simulink model "sigdemo_large_STRONG_SIGNATURE"  (Simulink 8.4)
settings: Solver=FixedStepDiscrete  StartTime=0.0  StopTime=50.0  FixedStep=0.0001  RelTol=1e-3
undefined symbols (not defined in the file or in its folder): CheckValue, DefaultMode, ErrorMode, FALSE, Mode1, Mode1Cal, Mode2, Mode3, Mode3Cal, Mode4, Mode4Cal, Mode4Val, TRUE
settings Model: Creator=chrysler2  LastModifiedBy=Ben
settings DebuggingCC: CheckSSInitialOutputMsg=off  MergeDetectMultiDrivingBlocksExec=error  FcnCallInpInsideContextMsg=EnableAllAsWarning

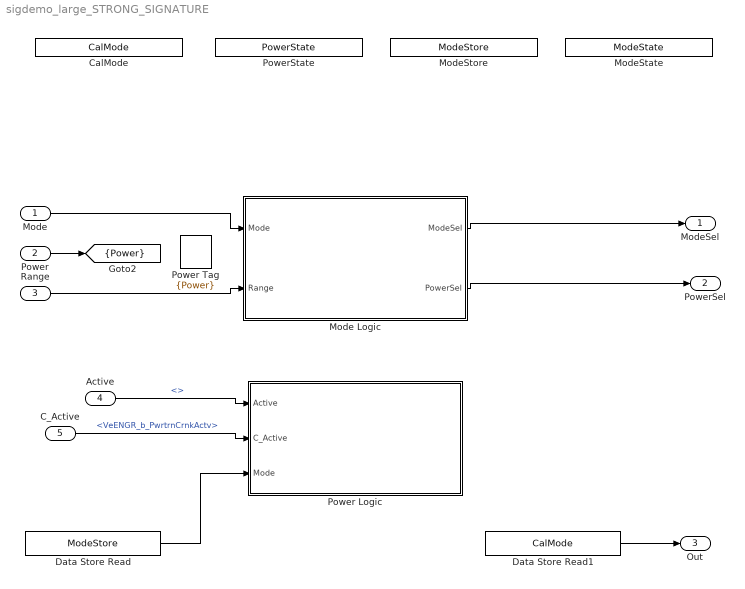
== system sigdemo_large_STRONG_SIGNATURE ==
  Mode : Inport
  Power : Inport  Port=2
  Range : Inport  Port=3
  Active : Inport  Port=4
  C_Active : Inport  Port=5
  CalMode : DataStoreMemory  DataStoreName=CalMode  OutDataTypeStr=uint16
  Data Store Read : DataStoreRead  DataStoreName=ModeStore
  Data Store Read1 : DataStoreRead  DataStoreName=CalMode
  Mode Logic : Subsystem
  ModeState : DataStoreMemory  DataStoreName=ModeState  OutDataTypeStr=uint16
  ModeStore : DataStoreMemory  DataStoreName=ModeStore  OutDataTypeStr=uint16
  Power Logic : Subsystem
  Power Tag : GotoTagVisibility  GotoTag=Power
  PowerState : DataStoreMemory  DataStoreName=PowerState  OutDataTypeStr=boolean
  ModeSel : Outport
  PowerSel : Outport  Port=2
  Out : Outport  Port=3
  tag scope: Power=scoped
  wires:
  Mode Logic/1(ModeSel) -> ModeSel/1
  Mode Logic/2(PowerSel) -> PowerSel/1
  Range/1 -> Mode Logic/2(Range)
  C_Active/1 -> Power Logic/2(C_Active)  "<VeENGR_b_PwrtrnCrnkActv>"
  Active/1 -> Power Logic/1(Active)  "<>"
  Mode/1 -> Mode Logic/1(Mode)
  Data Store Read/1 -> Power Logic/3(Mode)
  Data Store Read1/1 -> Out/1
  Power/1 -> [Power]

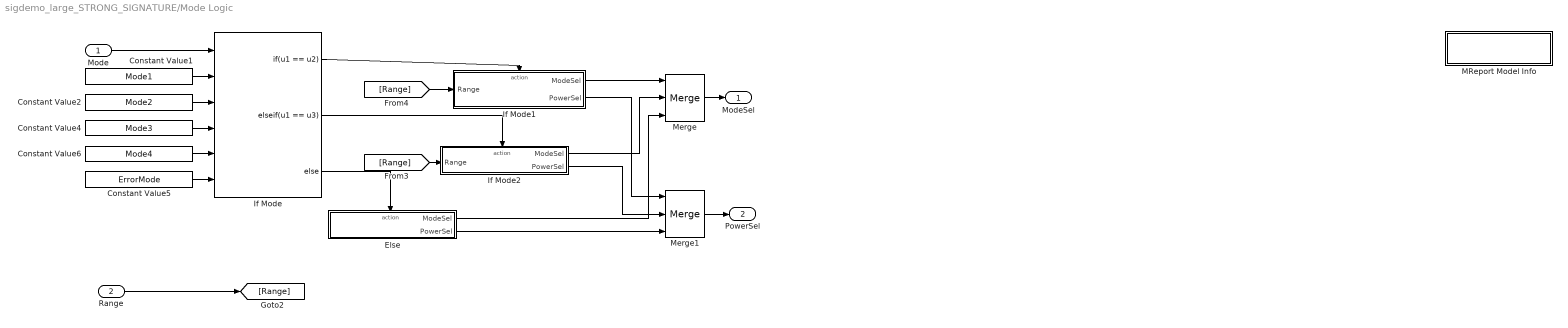
== system sigdemo_large_STRONG_SIGNATURE/Mode Logic ==
  Mode : Inport
  Range : Inport  Port=2
  Constant Value1 : Constant  Tag=R12-1  Value=Mode1  OutDataTypeStr=uint16  SampleTime=-1
  Constant Value2 : Constant  Tag=R12-1  Value=Mode2  OutDataTypeStr=uint16  SampleTime=-1
  Constant Value4 : Constant  Tag=R12-1  Value=Mode3  OutDataTypeStr=uint16  SampleTime=-1
  Constant Value5 : Constant  Tag=R12-1  Value=ErrorMode  OutDataTypeStr=uint16  SampleTime=-1
  Constant Value6 : Constant  Tag=R12-1  Value=Mode4  OutDataTypeStr=uint16  SampleTime=-1
  Else : Subsystem  TreatAsAtomicUnit=on
  If Mode : If  NumInputs=6  IfExpression=u1 == u2  ElseIfExpressions=u1 == u3
  If Mode1 : Subsystem  TreatAsAtomicUnit=on
  If Mode2 : Subsystem  TreatAsAtomicUnit=on
  MReport Model Info : Subsystem  mask(CMBlock){FollowLink=off, DocumentationField=|, HistoryField=, External=0}
      mask DocumentationField=|
      | This subsystem determines the desired neutral range state and desired engine state based on the PRNDL state.
      | The Drive functionality is executed when the PRNDL state is in DRIVE6 mode while the reverse functionality is triggered when PRNDL state is REVERSE. For other PRNDL states like Park, Neutral or Illegal the PNI functionality is executed.
      mask prompts: External "Mask Parameter 4:"
      mask help: This block allows to manage subsystem and history information.
      settings: OpenFcn=if isempty(which('mreport')),answer = char(inputdlg('Please define MReport path:'));addpath(answer);addpath([answer]);end;mr_model_info;
      mask Display: disp('MReport Model Info')
  Merge : Merge  Tag=R12-1  Inputs=3
  Merge1 : Merge  Tag=R12-1  Inputs=3
  ModeSel : Outport
  PowerSel : Outport  Port=2
  wires:
  [Range] -> If Mode2/1(Range)
  Mode/1 -> If Mode/1
  Constant Value1/1 -> If Mode/2
  Constant Value2/1 -> If Mode/3
  Constant Value4/1 -> If Mode/4
  Constant Value6/1 -> If Mode/5
  Constant Value5/1 -> If Mode/6
  If Mode/1 -> If Mode1/Action
  If Mode/3 -> Else/Action
  If Mode/2 -> If Mode2/Action
  Range/1 -> [Range]
  [Range] -> If Mode1/1(Range)
  If Mode1/1(ModeSel) -> Merge/1
  Merge/1 -> ModeSel/1
  Merge1/1 -> PowerSel/1
  If Mode1/2(PowerSel) -> Merge1/1
  If Mode2/1(ModeSel) -> Merge/2
  Else/1(ModeSel) -> Merge/3
  If Mode2/2(PowerSel) -> Merge1/2
  Else/2(PowerSel) -> Merge1/3

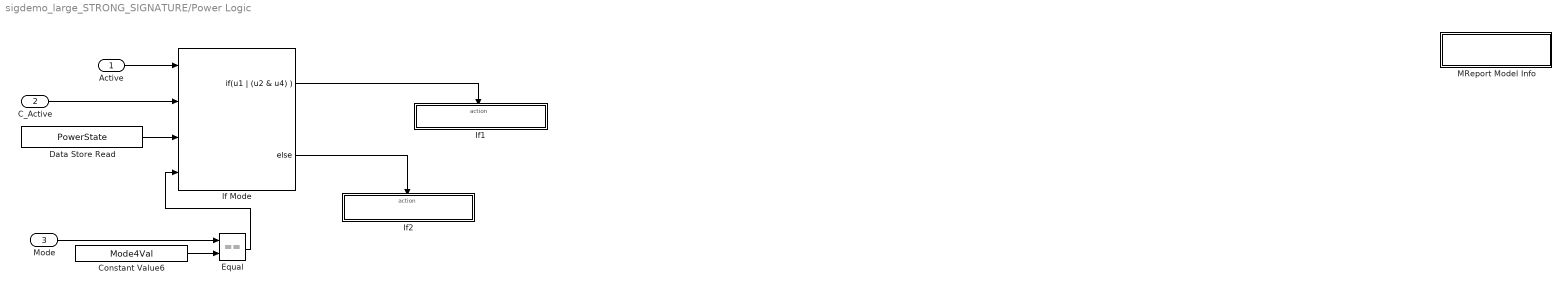
== system sigdemo_large_STRONG_SIGNATURE/Power Logic ==
  Active : Inport
  C_Active : Inport  Port=2
  Mode : Inport  Port=3
  Constant Value6 : Constant  Tag=R12-1  Value=Mode4Val  OutDataTypeStr=uint16  SampleTime=-1
  Data Store Read : DataStoreRead  DataStoreName=PowerState
  Equal : RelationalOperator  Tag=R12-1  Operator===  OutDataTypeStr=boolean  InputSameDT=on
  If Mode : If  NumInputs=4  IfExpression=u1 | (u2 & u4)
  If1 : Subsystem  TreatAsAtomicUnit=on
  If2 : Subsystem  TreatAsAtomicUnit=on
  MReport Model Info : Subsystem  mask(CMBlock){FollowLink=off, DocumentationField=|, HistoryField=, External=0}
      mask DocumentationField=|
      | This subsystem updates the following based on Gear Range state, Crank Now status, Power status and PT Active status:
      | a) Power On Timer Value
      | b) Power On Cold True Status
      | c) Power Status
      | d) Power On Cold Cost value
      |
      | The Power On functionality is triggered when PT is active or Cranking is enabled and Gear Range is in Parking or Neutral state otherwise the Power Off functionality is enabled to disable the Power status and updates Gear Range state by the Clutch Park or Neutral state. The Current Entry functionality is executed when the Power status is enabled.
      mask prompts: External "Mask Parameter 4:"
      mask help: This block allows to manage subsystem and history information.
      settings: OpenFcn=if isempty(which('mreport')),answer = char(inputdlg('Please define MReport path:'));addpath(answer);addpath([answer]);end;mr_model_info;
      mask Display: disp('MReport Model Info')
  wires:
  If Mode/2 -> If2/Action
  If Mode/1 -> If1/Action
  Active/1 -> If Mode/1
  C_Active/1 -> If Mode/2
  Data Store Read/1 -> If Mode/3
  Mode/1 -> Equal/1
  Constant Value6/1 -> Equal/2
  Equal/1 -> If Mode/4

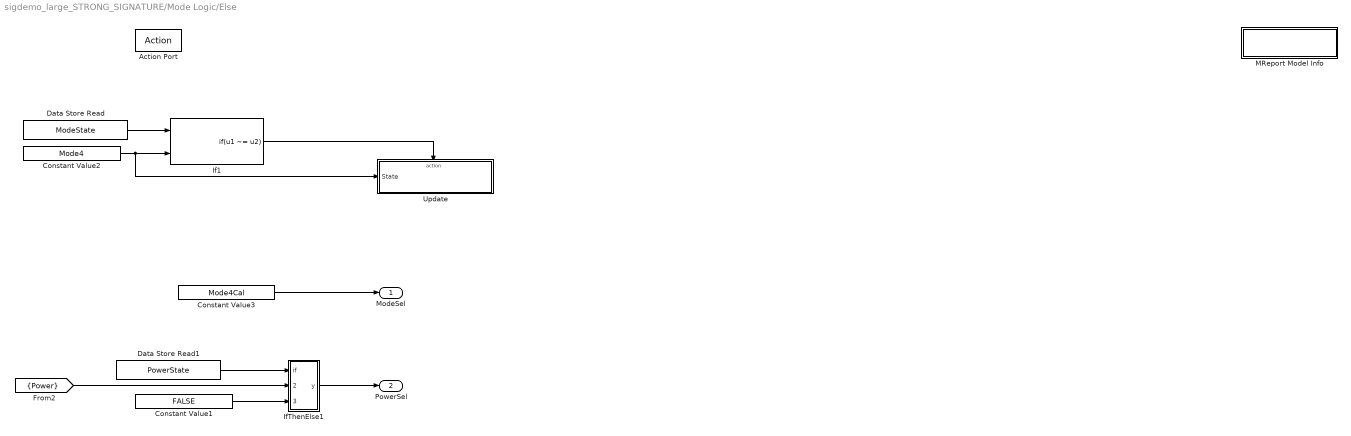
== system sigdemo_large_STRONG_SIGNATURE/Mode Logic/Else ==
  Action Port : ActionPort
  Constant Value1 : Constant  Tag=R12-1  Value=FALSE  OutDataTypeStr=boolean  SampleTime=-1
  Constant Value2 : Constant  Tag=R12-1  Value=Mode4  OutDataTypeStr=uint16  SampleTime=-1
  Constant Value3 : Constant  Tag=R12-1  Value=Mode4Cal  OutDataTypeStr=uint16  SampleTime=-1
  Data Store Read : DataStoreRead  DataStoreName=ModeState
  Data Store Read1 : DataStoreRead  DataStoreName=PowerState
  If1 : If  NumInputs=2  IfExpression=u1 ~= u2  ShowElse=off
  IfThenElse1 : Subsystem  Tag=R12-1  mask(IfElseif){}
      mask help: Output signal(s) will equal "then" values when "if" is TRUE, or hold their values if FALSE. Multiple signals can be pass by vectorizing the signals through the use of a mux block. Input1=IF condtion; Input2=IF action; Input3=ELSE action.
      mask Help: web(char(which([char(get_param(gcb,'MaskType')),'.html'])));
  MReport Model Info : Subsystem  mask(CMBlock){FollowLink=off, DocumentationField=|, HistoryField=, External=0}
      mask DocumentationField=|
      | This subsystem updates the following:
      | 1. State of Gear Range State by the PRNDL NEUTRAL state, Gear Range state by the Clutch Park or Neutral state. The Current Entry functionality is executed when the Gear Range State is not in PRNDL NEUTRAL state.
      | 2. Desired Neutral Range state by the Neutral Range Selection state.
      | 3. Desired Engine Selection indication by the Engine Selection indication or disables it depending upon Power Status.
      mask prompts: External "Mask Parameter 4:"
      mask help: This block allows to manage subsystem and history information.
      settings: OpenFcn=if isempty(which('mreport')),answer = char(inputdlg('Please define MReport path:'));addpath(answer);addpath([answer]);end;mr_model_info;
      mask Display: disp('MReport Model Info')
  Update : Subsystem  TreatAsAtomicUnit=on
  ModeSel : Outport
  PowerSel : Outport  Port=2
  wires:
  Data Store Read/1 -> If1/1
  If1/1 -> Update/Action
  Constant Value2/1 -> Update/1(State), If1/2
  IfThenElse1/1(y) -> PowerSel/1
  Data Store Read1/1 -> IfThenElse1/1(if)
  Constant Value1/1 -> IfThenElse1/3(else)
  Constant Value3/1 -> ModeSel/1
  [Power] -> IfThenElse1/2(then)

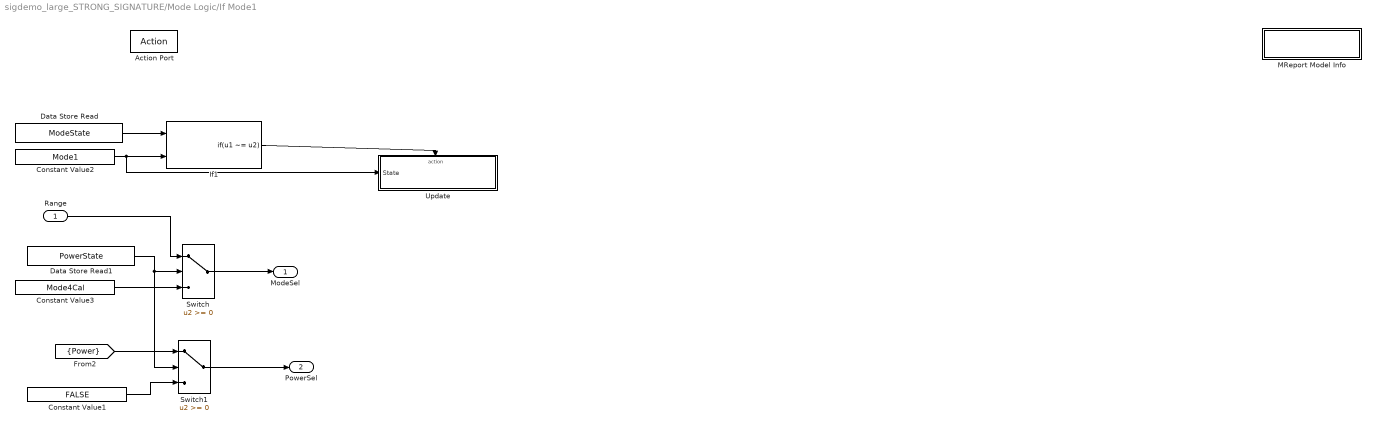
== system sigdemo_large_STRONG_SIGNATURE/Mode Logic/If Mode1 ==
  Range : Inport
  Action Port : ActionPort
  Constant Value1 : Constant  Tag=R12-1  Value=FALSE  OutDataTypeStr=boolean  SampleTime=-1
  Constant Value2 : Constant  Tag=R12-1  Value=Mode1  OutDataTypeStr=uint16  SampleTime=-1
  Constant Value3 : Constant  Tag=R12-1  Value=Mode4Cal  OutDataTypeStr=uint16  SampleTime=-1
  Data Store Read : DataStoreRead  DataStoreName=ModeState
  Data Store Read1 : DataStoreRead  DataStoreName=PowerState
  If1 : If  NumInputs=2  IfExpression=u1 ~= u2  ShowElse=off
  MReport Model Info : Subsystem  mask(CMBlock){FollowLink=off, DocumentationField=|, HistoryField=, External=0}
      mask DocumentationField=|
      | This subsystem updates the following:
      | 1. State of Gear Range State by the PRNDL DRIVE6 state and Gear Range state by the Clutch Drive state.The Current Entry functionality is executed when the Gear Range State is not in PRNDL DRIVE6 state.
      | 2. Desired Neutral Range state by the  Selection Range state or by Neutral Range Selection state based on Power Status.
      | 3. Desired Engine Selection indication by  Engine Selection indication or disables it based on Power Status.
      mask prompts: External "Mask Parameter 4:"
      mask help: This block allows to manage subsystem and history information.
      settings: OpenFcn=if isempty(which('mreport')),answer = char(inputdlg('Please define MReport path:'));addpath(answer);addpath([answer]);end;mr_model_info;
      mask Display: disp('MReport Model Info')
  Switch : Switch
  Switch1 : Switch
  Update : Subsystem  TreatAsAtomicUnit=on
  ModeSel : Outport
  PowerSel : Outport  Port=2
  wires:
  Data Store Read/1 -> If1/1
  If1/1 -> Update/Action
  Constant Value2/1 -> If1/2, Update/1(State)
  Switch/1 -> ModeSel/1
  Switch1/1 -> PowerSel/1
  Data Store Read1/1 -> Switch/2, Switch1/2
  Constant Value1/1 -> Switch1/3
  Constant Value3/1 -> Switch/3
  Range/1 -> Switch/1
  [Power] -> Switch1/1

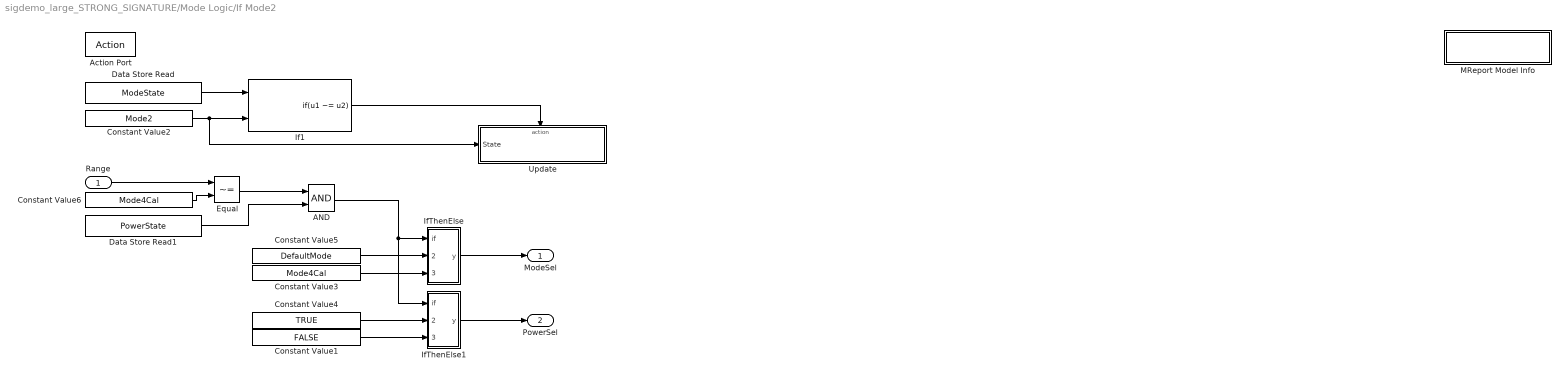
== system sigdemo_large_STRONG_SIGNATURE/Mode Logic/If Mode2 ==
  Range : Inport
  Action Port : ActionPort
  AND : Logic  Tag=R12-1  OutDataTypeStr=boolean
  Constant Value1 : Constant  Tag=R12-1  Value=FALSE  OutDataTypeStr=boolean  SampleTime=-1
  Constant Value2 : Constant  Tag=R12-1  Value=Mode2  OutDataTypeStr=uint16  SampleTime=-1
  Constant Value3 : Constant  Tag=R12-1  Value=Mode4Cal  OutDataTypeStr=uint16  SampleTime=-1
  Constant Value4 : Constant  Tag=R12-1  Value=TRUE  OutDataTypeStr=boolean  SampleTime=-1
  Constant Value5 : Constant  Tag=R12-1  Value=DefaultMode  OutDataTypeStr=uint16  SampleTime=-1
  Constant Value6 : Constant  Tag=R12-1  Value=Mode4Cal  OutDataTypeStr=uint16  SampleTime=-1
  Data Store Read : DataStoreRead  DataStoreName=ModeState
  Data Store Read1 : DataStoreRead  DataStoreName=PowerState
  Equal : RelationalOperator  Tag=R12-1  Operator=~=  OutDataTypeStr=boolean
  If1 : If  NumInputs=2  IfExpression=u1 ~= u2  ShowElse=off
  IfThenElse : Subsystem  Tag=R12-1  mask(IfElseif){}
      mask help: Output signal(s) will equal "then" values when "if" is TRUE, or hold their values if FALSE. Multiple signals can be pass by vectorizing the signals through the use of a mux block. Input1=IF condtion; Input2=IF action; Input3=ELSE action.
      mask Help: web(char(which([char(get_param(gcb,'MaskType')),'.html'])));
  IfThenElse1 : Subsystem  Tag=R12-1  mask(IfElseif){}
      mask help: Output signal(s) will equal "then" values when "if" is TRUE, or hold their values if FALSE. Multiple signals can be pass by vectorizing the signals through the use of a mux block. Input1=IF condtion; Input2=IF action; Input3=ELSE action.
      mask Help: web(char(which([char(get_param(gcb,'MaskType')),'.html'])));
  MReport Model Info : Subsystem  mask(CMBlock){FollowLink=off, DocumentationField=|, HistoryField=, External=0}
      mask DocumentationField=|
      | This subsystem performs the following:
      | 1. Updates state of Gear Range State by the PRNDL REVERSE state and Gear Range state by the Clutch Reverse state. The Current Entry functionality is executed when the Gear Range State is not in PRNDL REVERSE state.
      | 2. Updates Desired Neutral Range state by Mode 1 Range Selection state or by Neutral Range Selection state depending upon whether the value of Transmission Range Selection state is not in Neutral state and Power Status in active.
      | 3. Enables or Disables the Desired Engine Selection indication depending upon whether the value of  Transmission Range Selection state is not in Neutral state and Power Status in active.
      mask prompts: External "Mask Parameter 4:"
      mask help: This block allows to manage subsystem and history information.
      settings: OpenFcn=if isempty(which('mreport')),answer = char(inputdlg('Please define MReport path:'));addpath(answer);addpath([answer]);end;mr_model_info;
      mask Display: disp('MReport Model Info')
  Update : Subsystem  TreatAsAtomicUnit=on
  ModeSel : Outport
  PowerSel : Outport  Port=2
  wires:
  AND/1 -> IfThenElse/1(if), IfThenElse1/1(if)
  Data Store Read1/1 -> AND/2
  Equal/1 -> AND/1
  Constant Value6/1 -> Equal/2
  Range/1 -> Equal/1
  Constant Value2/1 -> If1/2, Update/1(State)
  If1/1 -> Update/Action
  Data Store Read/1 -> If1/1
  IfThenElse/1(y) -> ModeSel/1
  IfThenElse1/1(y) -> PowerSel/1
  Constant Value1/1 -> IfThenElse1/3(else)
  Constant Value3/1 -> IfThenElse/3(else)
  Constant Value4/1 -> IfThenElse1/2(then)
  Constant Value5/1 -> IfThenElse/2(then)

== system sigdemo_large_STRONG_SIGNATURE/Mode Logic/MReport Model Info ==
  EmptySubsystem : Subsystem

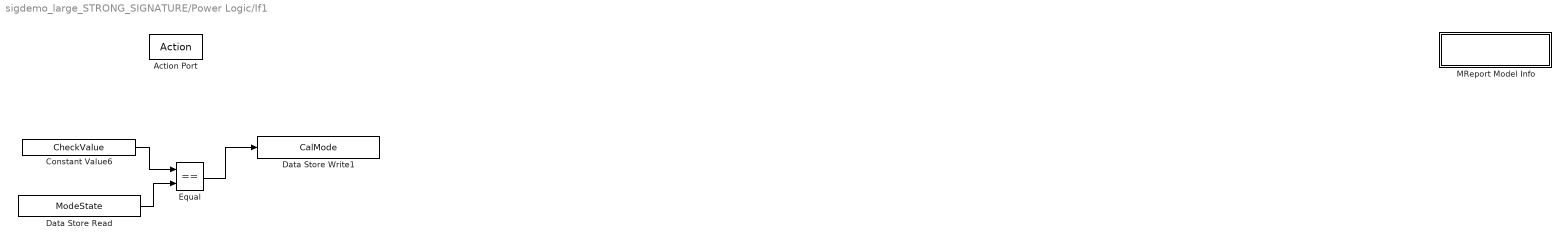
== system sigdemo_large_STRONG_SIGNATURE/Power Logic/If1 ==
  Action Port : ActionPort
  Constant Value6 : Constant  Tag=R12-1  Value=CheckValue  OutDataTypeStr=uint16  SampleTime=-1
  Data Store Read : DataStoreRead  DataStoreName=ModeState
  Data Store Write1 : DataStoreWrite  DataStoreName=CalMode
  Equal : RelationalOperator  Tag=R12-1  Operator===  OutDataTypeStr=boolean  InputSameDT=on
  MReport Model Info : Subsystem  mask(CMBlock){FollowLink=off, DocumentationField=|, HistoryField=, External=0}
      mask DocumentationField=|
      | This subsystem updates the following based on  Power status and Power On Cold True status:
      | a) Power On Timer Value
      | b) Power On Cold True Status
      | c) Power Status
      | d) Power On Cold Cost value
      | These parameters are updated using following functionalities:
      | a) The Current Entry functionality is executed when the Power Status is not in Active. It enables Power status, disables Power On Timer value and enables Power On Cold True status.
      | b) "During Cold" functionality is triggered when Power On Cold True Status is in active.
      | c) During Warm functionality is enabled when none of the above conditions are active and updates Power On Cold Cost value by KaHRSR_k_InitZero1x7.
      mask prompts: External "Mask Parameter 4:"
      mask help: This block allows to manage subsystem and history information.
      settings: OpenFcn=if isempty(which('mreport')),answer = char(inputdlg('Please define MReport path:'));addpath(answer);addpath([answer]);end;mr_model_info;
      mask Display: disp('MReport Model Info')
  wires:
  Constant Value6/1 -> Equal/1
  Data Store Read/1 -> Equal/2
  Equal/1 -> Data Store Write1/1

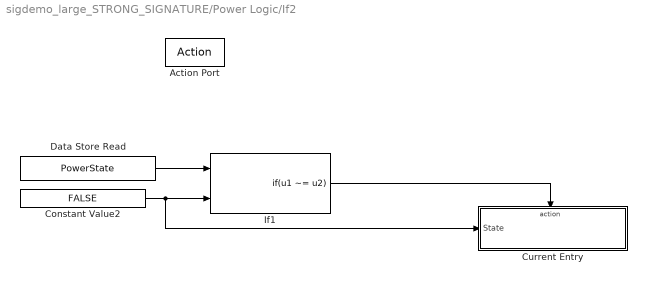
== system sigdemo_large_STRONG_SIGNATURE/Power Logic/If2 ==
  Action Port : ActionPort
  Constant Value2 : Constant  Tag=R12-1  Value=FALSE  OutDataTypeStr=boolean  SampleTime=-1
  Current Entry : Subsystem  TreatAsAtomicUnit=on
  Data Store Read : DataStoreRead  DataStoreName=PowerState
  If1 : If  NumInputs=2  IfExpression=u1 ~= u2  ShowElse=off
  wires:
  Constant Value2/1 -> If1/2, Current Entry/1(State)
  If1/1 -> Current Entry/Action
  Data Store Read/1 -> If1/1

== system sigdemo_large_STRONG_SIGNATURE/Power Logic/MReport Model Info ==
  EmptySubsystem : Subsystem

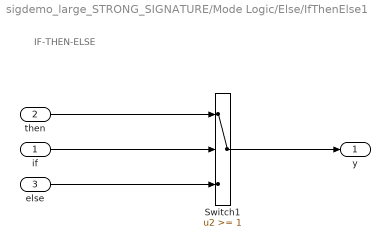
== system sigdemo_large_STRONG_SIGNATURE/Mode Logic/Else/IfThenElse1 ==
  note: IF-THEN-ELSE
  if : Inport  OutDataTypeStr=boolean
  then : Inport  Port=2
  else : Inport  Port=3
  Switch1 : Switch  Threshold=1  RndMeth=Zero  InputSameDT=on
      settings: AttributesFormatString=Threshold=%<Threshold>
  y : Outport
  wires:
  if/1 -> Switch1/2
  then/1 -> Switch1/1
  Switch1/1 -> y/1
  else/1 -> Switch1/3

== system sigdemo_large_STRONG_SIGNATURE/Mode Logic/Else/MReport Model Info ==
  EmptySubsystem : Subsystem

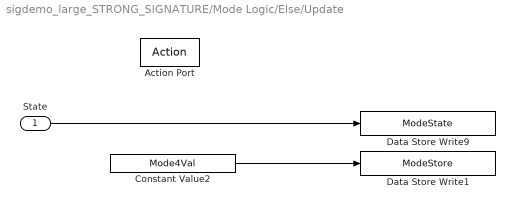
== system sigdemo_large_STRONG_SIGNATURE/Mode Logic/Else/Update ==
  State : Inport
  Action Port : ActionPort
  Constant Value2 : Constant  Tag=R12-1  Value=Mode4Val  OutDataTypeStr=uint16  SampleTime=-1
  Data Store Write1 : DataStoreWrite  DataStoreName=ModeStore
  Data Store Write9 : DataStoreWrite  DataStoreName=ModeState
  wires:
  State/1 -> Data Store Write9/1
  Constant Value2/1 -> Data Store Write1/1

== system sigdemo_large_STRONG_SIGNATURE/Mode Logic/If Mode1/MReport Model Info ==
  EmptySubsystem : Subsystem

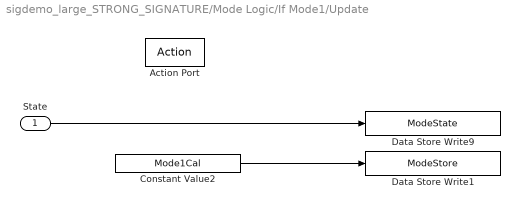
== system sigdemo_large_STRONG_SIGNATURE/Mode Logic/If Mode1/Update ==
  State : Inport
  Action Port : ActionPort
  Constant Value2 : Constant  Tag=R12-1  Value=Mode1Cal  OutDataTypeStr=uint16  SampleTime=-1
  Data Store Write1 : DataStoreWrite  DataStoreName=ModeStore
  Data Store Write9 : DataStoreWrite  DataStoreName=ModeState
  wires:
  Constant Value2/1 -> Data Store Write1/1
  State/1 -> Data Store Write9/1

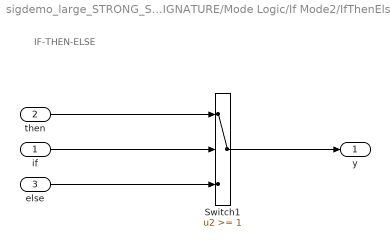
== system sigdemo_large_STRONG_SIGNATURE/Mode Logic/If Mode2/IfThenElse ==
  note: IF-THEN-ELSE
  if : Inport  OutDataTypeStr=boolean
  then : Inport  Port=2
  else : Inport  Port=3
  Switch1 : Switch  Threshold=1  RndMeth=Zero  InputSameDT=on
      settings: AttributesFormatString=Threshold=%<Threshold>
  y : Outport
  wires:
  if/1 -> Switch1/2
  then/1 -> Switch1/1
  Switch1/1 -> y/1
  else/1 -> Switch1/3

== system sigdemo_large_STRONG_SIGNATURE/Mode Logic/If Mode2/IfThenElse1 ==
  note: IF-THEN-ELSE
  if : Inport  OutDataTypeStr=boolean
  then : Inport  Port=2
  else : Inport  Port=3
  Switch1 : Switch  Threshold=1  RndMeth=Zero  InputSameDT=on
      settings: AttributesFormatString=Threshold=%<Threshold>
  y : Outport
  wires:
  if/1 -> Switch1/2
  then/1 -> Switch1/1
  Switch1/1 -> y/1
  else/1 -> Switch1/3

== system sigdemo_large_STRONG_SIGNATURE/Mode Logic/If Mode2/MReport Model Info ==
  EmptySubsystem : Subsystem

== system sigdemo_large_STRONG_SIGNATURE/Mode Logic/If Mode2/Update ==
  State : Inport
  Action Port : ActionPort
  Constant Value2 : Constant  Tag=R12-1  Value=Mode3Cal  OutDataTypeStr=uint16  SampleTime=-1
  Data Store Write1 : DataStoreWrite  DataStoreName=ModeStore
  Data Store Write9 : DataStoreWrite  DataStoreName=ModeState
  wires:
  Constant Value2/1 -> Data Store Write1/1
  State/1 -> Data Store Write9/1

== system sigdemo_large_STRONG_SIGNATURE/Mode Logic/MReport Model Info/EmptySubsystem ==

== system sigdemo_large_STRONG_SIGNATURE/Power Logic/If1/MReport Model Info ==
  EmptySubsystem : Subsystem

== system sigdemo_large_STRONG_SIGNATURE/Power Logic/If2/Current Entry ==
  State : Inport
  Action Port : ActionPort
  Constant Value2 : Constant  Tag=R12-1  Value=Mode4Val  OutDataTypeStr=uint16  SampleTime=-1
  Data Store Write1 : DataStoreWrite  DataStoreName=ModeStore
  Data Store Write9 : DataStoreWrite  DataStoreName=PowerState
  wires:
  Constant Value2/1 -> Data Store Write1/1
  State/1 -> Data Store Write9/1

== system sigdemo_large_STRONG_SIGNATURE/Power Logic/MReport Model Info/EmptySubsystem ==

== system sigdemo_large_STRONG_SIGNATURE/Mode Logic/Else/MReport Model Info/EmptySubsystem ==

== system sigdemo_large_STRONG_SIGNATURE/Mode Logic/If Mode1/MReport Model Info/EmptySubsystem ==

== system sigdemo_large_STRONG_SIGNATURE/Mode Logic/If Mode2/MReport Model Info/EmptySubsystem ==

== system sigdemo_large_STRONG_SIGNATURE/Power Logic/If1/MReport Model Info/EmptySubsystem ==
